simulink model "c00001M_harness"  (R2018a)
settings: Solver=ode3  StartTime=0.0  StopTime=10.0  RelTol=1e-3  EnableMultiTasking=on
undefined symbols (not defined in the file): b, DiscIntNeverNeededParam, J, K, L, R, sigbuilder_block
(part 4 of 19)

== system c00001M_harness/M084 ==
  DW1 : Inport  OutMin=0  OutMax=4  OutDataTypeStr=int8
  P1W2 : Inport  Port=2  OutMin=0  OutMax=4  OutDataTypeStr=int8
  O1 : Inport  Port=3  OutDataTypeStr=boolean
  O2 : Inport  Port=4  OutDataTypeStr=boolean
  Cyber : Subsystem
  M : Memory
  M1 : Memory
  Physical : Subsystem
  S1 : Subsystem
  S2 : Subsystem
  W1Pos : Outport
  W2Pos : Outport  Port=2
  wires:
  S2/1(SensorOut) -> M1/1
  Physical/2(W2) -> S2/1(PhyMeasure), W2Pos/1
  DW1/1 -> Cyber/3(DW1)
  M/1 -> Cyber/1(PosW1)
  M1/1 -> Cyber/2(PosW2)
  P1W2/1 -> Cyber/4(P1W2)
  Cyber/2(W2) -> Physical/2(InW2)
  Cyber/1(W1) -> Physical/1(InW1)
  O1/1 -> Cyber/5(OW1)
  O2/1 -> Cyber/6(OW2)
  Physical/1(W1) -> S1/1(PhyMeasure), W1Pos/1
  S1/1(SensorOut) -> M/1

== system c00001M_harness/M087 ==
  DW1 : Inport  OutMin=0  OutMax=4  OutDataTypeStr=int8
  P1W2 : Inport  Port=2  OutMin=0  OutMax=4  OutDataTypeStr=int8
  O1 : Inport  Port=3  OutDataTypeStr=boolean
  O2 : Inport  Port=4  OutDataTypeStr=boolean
  Cyber : Subsystem
  M : Memory
  M1 : Memory
  Physical : Subsystem
  S1 : Subsystem
  S2 : Subsystem
  W1Pos : Outport
  W2Pos : Outport  Port=2
  wires:
  S2/1(SensorOut) -> M1/1
  Physical/2(W2) -> S2/1(PhyMeasure), W2Pos/1
  DW1/1 -> Cyber/3(DW1)
  M/1 -> Cyber/1(PosW1)
  M1/1 -> Cyber/2(PosW2)
  P1W2/1 -> Cyber/4(P1W2)
  Cyber/2(W2) -> Physical/2(InW2)
  Cyber/1(W1) -> Physical/1(InW1)
  O1/1 -> Cyber/5(OW1)
  O2/1 -> Cyber/6(OW2)
  Physical/1(W1) -> S1/1(PhyMeasure), W1Pos/1
  S1/1(SensorOut) -> M/1

== system c00001M_harness/M088 ==
  DW1 : Inport  OutMin=0  OutMax=4  OutDataTypeStr=int8
  P1W2 : Inport  Port=2  OutMin=0  OutMax=4  OutDataTypeStr=int8
  O1 : Inport  Port=3  OutDataTypeStr=boolean
  O2 : Inport  Port=4  OutDataTypeStr=boolean
  Cyber : Subsystem
  M : Memory
  M1 : Memory
  Physical : Subsystem
  S1 : Subsystem
  S2 : Subsystem
  W1Pos : Outport
  W2Pos : Outport  Port=2
  wires:
  S2/1(SensorOut) -> M1/1
  Physical/2(W2) -> S2/1(PhyMeasure), W2Pos/1
  DW1/1 -> Cyber/3(DW1)
  M/1 -> Cyber/1(PosW1)
  M1/1 -> Cyber/2(PosW2)
  P1W2/1 -> Cyber/4(P1W2)
  Cyber/2(W2) -> Physical/2(InW2)
  Cyber/1(W1) -> Physical/1(InW1)
  O1/1 -> Cyber/5(OW1)
  O2/1 -> Cyber/6(OW2)
  Physical/1(W1) -> S1/1(PhyMeasure), W1Pos/1
  S1/1(SensorOut) -> M/1

== system c00001M_harness/M091 ==
  DW1 : Inport  OutMin=0  OutMax=4  OutDataTypeStr=int8
  P1W2 : Inport  Port=2  OutMin=0  OutMax=4  OutDataTypeStr=int8
  O1 : Inport  Port=3  OutDataTypeStr=boolean
  O2 : Inport  Port=4  OutDataTypeStr=boolean
  Cyber : Subsystem
  M : Memory
  M1 : Memory
  Physical : Subsystem
  S1 : Subsystem
  S2 : Subsystem
  W1Pos : Outport
  W2Pos : Outport  Port=2
  wires:
  S2/1(SensorOut) -> M1/1
  Physical/2(W2) -> S2/1(PhyMeasure), W2Pos/1
  DW1/1 -> Cyber/3(DW1)
  M/1 -> Cyber/1(PosW1)
  M1/1 -> Cyber/2(PosW2)
  P1W2/1 -> Cyber/4(P1W2)
  Cyber/2(W2) -> Physical/2(InW2)
  Cyber/1(W1) -> Physical/1(InW1)
  O1/1 -> Cyber/5(OW1)
  O2/1 -> Cyber/6(OW2)
  Physical/1(W1) -> S1/1(PhyMeasure), W1Pos/1
  S1/1(SensorOut) -> M/1

== system c00001M_harness/M092 ==
  DW1 : Inport  OutMin=0  OutMax=4  OutDataTypeStr=int8
  P1W2 : Inport  Port=2  OutMin=0  OutMax=4  OutDataTypeStr=int8
  O1 : Inport  Port=3  OutDataTypeStr=boolean
  O2 : Inport  Port=4  OutDataTypeStr=boolean
  Cyber : Subsystem
  M : Memory
  M1 : Memory
  Physical : Subsystem
  S1 : Subsystem
  S2 : Subsystem
  W1Pos : Outport
  W2Pos : Outport  Port=2
  wires:
  S2/1(SensorOut) -> M1/1
  Physical/2(W2) -> S2/1(PhyMeasure), W2Pos/1
  DW1/1 -> Cyber/3(DW1)
  M/1 -> Cyber/1(PosW1)
  M1/1 -> Cyber/2(PosW2)
  P1W2/1 -> Cyber/4(P1W2)
  Cyber/2(W2) -> Physical/2(InW2)
  Cyber/1(W1) -> Physical/1(InW1)
  O1/1 -> Cyber/5(OW1)
  O2/1 -> Cyber/6(OW2)
  Physical/1(W1) -> S1/1(PhyMeasure), W1Pos/1
  S1/1(SensorOut) -> M/1

== system c00001M_harness/M095 ==
  DW1 : Inport  OutMin=0  OutMax=4  OutDataTypeStr=int8
  P1W2 : Inport  Port=2  OutMin=0  OutMax=4  OutDataTypeStr=int8
  O1 : Inport  Port=3  OutDataTypeStr=boolean
  O2 : Inport  Port=4  OutDataTypeStr=boolean
  Cyber : Subsystem
  M : Memory
  M1 : Memory
  Physical : Subsystem
  S1 : Subsystem
  S2 : Subsystem
  W1Pos : Outport
  W2Pos : Outport  Port=2
  wires:
  S2/1(SensorOut) -> M1/1
  Physical/2(W2) -> S2/1(PhyMeasure), W2Pos/1
  DW1/1 -> Cyber/3(DW1)
  M/1 -> Cyber/1(PosW1)
  M1/1 -> Cyber/2(PosW2)
  P1W2/1 -> Cyber/4(P1W2)
  Cyber/2(W2) -> Physical/2(InW2)
  Cyber/1(W1) -> Physical/1(InW1)
  O1/1 -> Cyber/5(OW1)
  O2/1 -> Cyber/6(OW2)
  Physical/1(W1) -> S1/1(PhyMeasure), W1Pos/1
  S1/1(SensorOut) -> M/1

== system c00001M_harness/M096 ==
  DW1 : Inport  OutMin=0  OutMax=4  OutDataTypeStr=int8
  P1W2 : Inport  Port=2  OutMin=0  OutMax=4  OutDataTypeStr=int8
  O1 : Inport  Port=3  OutDataTypeStr=boolean
  O2 : Inport  Port=4  OutDataTypeStr=boolean
  Cyber : Subsystem
  M : Memory
  M1 : Memory
  Physical : Subsystem
  S1 : Subsystem
  S2 : Subsystem
  W1Pos : Outport
  W2Pos : Outport  Port=2
  wires:
  S2/1(SensorOut) -> M1/1
  Physical/2(W2) -> S2/1(PhyMeasure), W2Pos/1
  DW1/1 -> Cyber/3(DW1)
  M/1 -> Cyber/1(PosW1)
  M1/1 -> Cyber/2(PosW2)
  P1W2/1 -> Cyber/4(P1W2)
  Cyber/2(W2) -> Physical/2(InW2)
  Cyber/1(W1) -> Physical/1(InW1)
  O1/1 -> Cyber/5(OW1)
  O2/1 -> Cyber/6(OW2)
  Physical/1(W1) -> S1/1(PhyMeasure), W1Pos/1
  S1/1(SensorOut) -> M/1

== system c00001M_harness/M099 ==
  DW1 : Inport  OutMin=0  OutMax=4  OutDataTypeStr=int8
  P1W2 : Inport  Port=2  OutMin=0  OutMax=4  OutDataTypeStr=int8
  O1 : Inport  Port=3  OutDataTypeStr=boolean
  O2 : Inport  Port=4  OutDataTypeStr=boolean
  Cyber : Subsystem
  M : Memory
  M1 : Memory
  Physical : Subsystem
  S1 : Subsystem
  S2 : Subsystem
  W1Pos : Outport
  W2Pos : Outport  Port=2
  wires:
  S2/1(SensorOut) -> M1/1
  Physical/2(W2) -> S2/1(PhyMeasure), W2Pos/1
  DW1/1 -> Cyber/3(DW1)
  M/1 -> Cyber/1(PosW1)
  M1/1 -> Cyber/2(PosW2)
  P1W2/1 -> Cyber/4(P1W2)
  Cyber/2(W2) -> Physical/2(InW2)
  Cyber/1(W1) -> Physical/1(InW1)
  O1/1 -> Cyber/5(OW1)
  O2/1 -> Cyber/6(OW2)
  Physical/1(W1) -> S1/1(PhyMeasure), W1Pos/1
  S1/1(SensorOut) -> M/1

== system c00001M_harness/M100 ==
  DW1 : Inport  OutMin=0  OutMax=4  OutDataTypeStr=int8
  P1W2 : Inport  Port=2  OutMin=0  OutMax=4  OutDataTypeStr=int8
  O1 : Inport  Port=3  OutDataTypeStr=boolean
  O2 : Inport  Port=4  OutDataTypeStr=boolean
  Cyber : Subsystem
  M : Memory
  M1 : Memory
  Physical : Subsystem
  S1 : Subsystem
  S2 : Subsystem
  W1Pos : Outport
  W2Pos : Outport  Port=2
  wires:
  S2/1(SensorOut) -> M1/1
  Physical/2(W2) -> S2/1(PhyMeasure), W2Pos/1
  DW1/1 -> Cyber/3(DW1)
  M/1 -> Cyber/1(PosW1)
  M1/1 -> Cyber/2(PosW2)
  P1W2/1 -> Cyber/4(P1W2)
  Cyber/2(W2) -> Physical/2(InW2)
  Cyber/1(W1) -> Physical/1(InW1)
  O1/1 -> Cyber/5(OW1)
  O2/1 -> Cyber/6(OW2)
  Physical/1(W1) -> S1/1(PhyMeasure), W1Pos/1
  S1/1(SensorOut) -> M/1

== system c00001M_harness/M103 ==
  DW1 : Inport  OutMin=0  OutMax=4  OutDataTypeStr=int8
  P1W2 : Inport  Port=2  OutMin=0  OutMax=4  OutDataTypeStr=int8
  O1 : Inport  Port=3  OutDataTypeStr=boolean
  O2 : Inport  Port=4  OutDataTypeStr=boolean
  Cyber : Subsystem
  M : Memory
  M1 : Memory
  Physical : Subsystem
  S1 : Subsystem
  S2 : Subsystem
  W1Pos : Outport
  W2Pos : Outport  Port=2
  wires:
  S2/1(SensorOut) -> M1/1
  Physical/2(W2) -> S2/1(PhyMeasure), W2Pos/1
  DW1/1 -> Cyber/3(DW1)
  M/1 -> Cyber/1(PosW1)
  M1/1 -> Cyber/2(PosW2)
  P1W2/1 -> Cyber/4(P1W2)
  Cyber/2(W2) -> Physical/2(InW2)
  Cyber/1(W1) -> Physical/1(InW1)
  O1/1 -> Cyber/5(OW1)
  O2/1 -> Cyber/6(OW2)
  Physical/1(W1) -> S1/1(PhyMeasure), W1Pos/1
  S1/1(SensorOut) -> M/1

== system c00001M_harness/M104 ==
  DW1 : Inport  OutMin=0  OutMax=4  OutDataTypeStr=int8
  P1W2 : Inport  Port=2  OutMin=0  OutMax=4  OutDataTypeStr=int8
  O1 : Inport  Port=3  OutDataTypeStr=boolean
  O2 : Inport  Port=4  OutDataTypeStr=boolean
  Cyber : Subsystem
  M : Memory
  M1 : Memory
  Physical : Subsystem
  S1 : Subsystem
  S2 : Subsystem
  W1Pos : Outport
  W2Pos : Outport  Port=2
  wires:
  S2/1(SensorOut) -> M1/1
  Physical/2(W2) -> S2/1(PhyMeasure), W2Pos/1
  DW1/1 -> Cyber/3(DW1)
  M/1 -> Cyber/1(PosW1)
  M1/1 -> Cyber/2(PosW2)
  P1W2/1 -> Cyber/4(P1W2)
  Cyber/2(W2) -> Physical/2(InW2)
  Cyber/1(W1) -> Physical/1(InW1)
  O1/1 -> Cyber/5(OW1)
  O2/1 -> Cyber/6(OW2)
  Physical/1(W1) -> S1/1(PhyMeasure), W1Pos/1
  S1/1(SensorOut) -> M/1

== system c00001M_harness/M107 ==
  DW1 : Inport  OutMin=0  OutMax=4  OutDataTypeStr=int8
  P1W2 : Inport  Port=2  OutMin=0  OutMax=4  OutDataTypeStr=int8
  O1 : Inport  Port=3  OutDataTypeStr=boolean
  O2 : Inport  Port=4  OutDataTypeStr=boolean
  Cyber : Subsystem
  M : Memory
  M1 : Memory
  Physical : Subsystem
  S1 : Subsystem
  S2 : Subsystem
  W1Pos : Outport
  W2Pos : Outport  Port=2
  wires:
  S2/1(SensorOut) -> M1/1
  Physical/2(W2) -> S2/1(PhyMeasure), W2Pos/1
  DW1/1 -> Cyber/3(DW1)
  M/1 -> Cyber/1(PosW1)
  M1/1 -> Cyber/2(PosW2)
  P1W2/1 -> Cyber/4(P1W2)
  Cyber/2(W2) -> Physical/2(InW2)
  Cyber/1(W1) -> Physical/1(InW1)
  O1/1 -> Cyber/5(OW1)
  O2/1 -> Cyber/6(OW2)
  Physical/1(W1) -> S1/1(PhyMeasure), W1Pos/1
  S1/1(SensorOut) -> M/1

== system c00001M_harness/M108 ==
  DW1 : Inport  OutMin=0  OutMax=4  OutDataTypeStr=int8
  P1W2 : Inport  Port=2  OutMin=0  OutMax=4  OutDataTypeStr=int8
  O1 : Inport  Port=3  OutDataTypeStr=boolean
  O2 : Inport  Port=4  OutDataTypeStr=boolean
  Cyber : Subsystem
  M : Memory
  M1 : Memory
  Physical : Subsystem
  S1 : Subsystem
  S2 : Subsystem
  W1Pos : Outport
  W2Pos : Outport  Port=2
  wires:
  S2/1(SensorOut) -> M1/1
  Physical/2(W2) -> S2/1(PhyMeasure), W2Pos/1
  DW1/1 -> Cyber/3(DW1)
  M/1 -> Cyber/1(PosW1)
  M1/1 -> Cyber/2(PosW2)
  P1W2/1 -> Cyber/4(P1W2)
  Cyber/2(W2) -> Physical/2(InW2)
  Cyber/1(W1) -> Physical/1(InW1)
  O1/1 -> Cyber/5(OW1)
  O2/1 -> Cyber/6(OW2)
  Physical/1(W1) -> S1/1(PhyMeasure), W1Pos/1
  S1/1(SensorOut) -> M/1

== system c00001M_harness/M111 ==
  DW1 : Inport  OutMin=0  OutMax=4  OutDataTypeStr=int8
  P1W2 : Inport  Port=2  OutMin=0  OutMax=4  OutDataTypeStr=int8
  O1 : Inport  Port=3  OutDataTypeStr=boolean
  O2 : Inport  Port=4  OutDataTypeStr=boolean
  Cyber : Subsystem
  M : Memory
  M1 : Memory
  Physical : Subsystem
  S1 : Subsystem
  S2 : Subsystem
  W1Pos : Outport
  W2Pos : Outport  Port=2
  wires:
  S2/1(SensorOut) -> M1/1
  Physical/2(W2) -> S2/1(PhyMeasure), W2Pos/1
  DW1/1 -> Cyber/3(DW1)
  M/1 -> Cyber/1(PosW1)
  M1/1 -> Cyber/2(PosW2)
  P1W2/1 -> Cyber/4(P1W2)
  Cyber/2(W2) -> Physical/2(InW2)
  Cyber/1(W1) -> Physical/1(InW1)
  O1/1 -> Cyber/5(OW1)
  O2/1 -> Cyber/6(OW2)
  Physical/1(W1) -> S1/1(PhyMeasure), W1Pos/1
  S1/1(SensorOut) -> M/1

== system c00001M_harness/M112 ==
  DW1 : Inport  OutMin=0  OutMax=4  OutDataTypeStr=int8
  P1W2 : Inport  Port=2  OutMin=0  OutMax=4  OutDataTypeStr=int8
  O1 : Inport  Port=3  OutDataTypeStr=boolean
  O2 : Inport  Port=4  OutDataTypeStr=boolean
  Cyber : Subsystem
  M : Memory
  M1 : Memory
  Physical : Subsystem
  S1 : Subsystem
  S2 : Subsystem
  W1Pos : Outport
  W2Pos : Outport  Port=2
  wires:
  S2/1(SensorOut) -> M1/1
  Physical/2(W2) -> S2/1(PhyMeasure), W2Pos/1
  DW1/1 -> Cyber/3(DW1)
  M/1 -> Cyber/1(PosW1)
  M1/1 -> Cyber/2(PosW2)
  P1W2/1 -> Cyber/4(P1W2)
  Cyber/2(W2) -> Physical/2(InW2)
  Cyber/1(W1) -> Physical/1(InW1)
  O1/1 -> Cyber/5(OW1)
  O2/1 -> Cyber/6(OW2)
  Physical/1(W1) -> S1/1(PhyMeasure), W1Pos/1
  S1/1(SensorOut) -> M/1

== system c00001M_harness/M115 ==
  DW1 : Inport  OutMin=0  OutMax=4  OutDataTypeStr=int8
  P1W2 : Inport  Port=2  OutMin=0  OutMax=4  OutDataTypeStr=int8
  O1 : Inport  Port=3  OutDataTypeStr=boolean
  O2 : Inport  Port=4  OutDataTypeStr=boolean
  Cyber : Subsystem
  M : Memory
  M1 : Memory
  Physical : Subsystem
  S1 : Subsystem
  S2 : Subsystem
  W1Pos : Outport
  W2Pos : Outport  Port=2
  wires:
  S2/1(SensorOut) -> M1/1
  Physical/2(W2) -> S2/1(PhyMeasure), W2Pos/1
  DW1/1 -> Cyber/3(DW1)
  M/1 -> Cyber/1(PosW1)
  M1/1 -> Cyber/2(PosW2)
  P1W2/1 -> Cyber/4(P1W2)
  Cyber/2(W2) -> Physical/2(InW2)
  Cyber/1(W1) -> Physical/1(InW1)
  O1/1 -> Cyber/5(OW1)
  O2/1 -> Cyber/6(OW2)
  Physical/1(W1) -> S1/1(PhyMeasure), W1Pos/1
  S1/1(SensorOut) -> M/1

== system c00001M_harness/M116 ==
  DW1 : Inport  OutMin=0  OutMax=4  OutDataTypeStr=int8
  P1W2 : Inport  Port=2  OutMin=0  OutMax=4  OutDataTypeStr=int8
  O1 : Inport  Port=3  OutDataTypeStr=boolean
  O2 : Inport  Port=4  OutDataTypeStr=boolean
  Cyber : Subsystem
  M : Memory
  M1 : Memory
  Physical : Subsystem
  S1 : Subsystem
  S2 : Subsystem
  W1Pos : Outport
  W2Pos : Outport  Port=2
  wires:
  S2/1(SensorOut) -> M1/1
  Physical/2(W2) -> S2/1(PhyMeasure), W2Pos/1
  DW1/1 -> Cyber/3(DW1)
  M/1 -> Cyber/1(PosW1)
  M1/1 -> Cyber/2(PosW2)
  P1W2/1 -> Cyber/4(P1W2)
  Cyber/2(W2) -> Physical/2(InW2)
  Cyber/1(W1) -> Physical/1(InW1)
  O1/1 -> Cyber/5(OW1)
  O2/1 -> Cyber/6(OW2)
  Physical/1(W1) -> S1/1(PhyMeasure), W1Pos/1
  S1/1(SensorOut) -> M/1

== system c00001M_harness/M119 ==
  DW1 : Inport  OutMin=0  OutMax=4  OutDataTypeStr=int8
  P1W2 : Inport  Port=2  OutMin=0  OutMax=4  OutDataTypeStr=int8
  O1 : Inport  Port=3  OutDataTypeStr=boolean
  O2 : Inport  Port=4  OutDataTypeStr=boolean
  Cyber : Subsystem
  M : Memory
  M1 : Memory
  Physical : Subsystem
  S1 : Subsystem
  S2 : Subsystem
  W1Pos : Outport
  W2Pos : Outport  Port=2
  wires:
  S2/1(SensorOut) -> M1/1
  Physical/2(W2) -> S2/1(PhyMeasure), W2Pos/1
  DW1/1 -> Cyber/3(DW1)
  M/1 -> Cyber/1(PosW1)
  M1/1 -> Cyber/2(PosW2)
  P1W2/1 -> Cyber/4(P1W2)
  Cyber/2(W2) -> Physical/2(InW2)
  Cyber/1(W1) -> Physical/1(InW1)
  O1/1 -> Cyber/5(OW1)
  O2/1 -> Cyber/6(OW2)
  Physical/1(W1) -> S1/1(PhyMeasure), W1Pos/1
  S1/1(SensorOut) -> M/1

== system c00001M_harness/M120 ==
  DW1 : Inport  OutMin=0  OutMax=4  OutDataTypeStr=int8
  P1W2 : Inport  Port=2  OutMin=0  OutMax=4  OutDataTypeStr=int8
  O1 : Inport  Port=3  OutDataTypeStr=boolean
  O2 : Inport  Port=4  OutDataTypeStr=boolean
  Cyber : Subsystem
  M : Memory
  M1 : Memory
  Physical : Subsystem
  S1 : Subsystem
  S2 : Subsystem
  W1Pos : Outport
  W2Pos : Outport  Port=2
  wires:
  S2/1(SensorOut) -> M1/1
  Physical/2(W2) -> S2/1(PhyMeasure), W2Pos/1
  DW1/1 -> Cyber/3(DW1)
  M/1 -> Cyber/1(PosW1)
  M1/1 -> Cyber/2(PosW2)
  P1W2/1 -> Cyber/4(P1W2)
  Cyber/2(W2) -> Physical/2(InW2)
  Cyber/1(W1) -> Physical/1(InW1)
  O1/1 -> Cyber/5(OW1)
  O2/1 -> Cyber/6(OW2)
  Physical/1(W1) -> S1/1(PhyMeasure), W1Pos/1
  S1/1(SensorOut) -> M/1

== system c00001M_harness/M123 ==
  DW1 : Inport  OutMin=0  OutMax=4  OutDataTypeStr=int8
  P1W2 : Inport  Port=2  OutMin=0  OutMax=4  OutDataTypeStr=int8
  O1 : Inport  Port=3  OutDataTypeStr=boolean
  O2 : Inport  Port=4  OutDataTypeStr=boolean
  Cyber : Subsystem
  M : Memory
  M1 : Memory
  Physical : Subsystem
  S1 : Subsystem
  S2 : Subsystem
  W1Pos : Outport
  W2Pos : Outport  Port=2
  wires:
  S2/1(SensorOut) -> M1/1
  Physical/2(W2) -> S2/1(PhyMeasure), W2Pos/1
  DW1/1 -> Cyber/3(DW1)
  M/1 -> Cyber/1(PosW1)
  M1/1 -> Cyber/2(PosW2)
  P1W2/1 -> Cyber/4(P1W2)
  Cyber/2(W2) -> Physical/2(InW2)
  Cyber/1(W1) -> Physical/1(InW1)
  O1/1 -> Cyber/5(OW1)
  O2/1 -> Cyber/6(OW2)
  Physical/1(W1) -> S1/1(PhyMeasure), W1Pos/1
  S1/1(SensorOut) -> M/1

== system c00001M_harness/M124 ==
  DW1 : Inport  OutMin=0  OutMax=4  OutDataTypeStr=int8
  P1W2 : Inport  Port=2  OutMin=0  OutMax=4  OutDataTypeStr=int8
  O1 : Inport  Port=3  OutDataTypeStr=boolean
  O2 : Inport  Port=4  OutDataTypeStr=boolean
  Cyber : Subsystem
  M : Memory
  M1 : Memory
  Physical : Subsystem
  S1 : Subsystem
  S2 : Subsystem
  W1Pos : Outport
  W2Pos : Outport  Port=2
  wires:
  S2/1(SensorOut) -> M1/1
  Physical/2(W2) -> S2/1(PhyMeasure), W2Pos/1
  DW1/1 -> Cyber/3(DW1)
  M/1 -> Cyber/1(PosW1)
  M1/1 -> Cyber/2(PosW2)
  P1W2/1 -> Cyber/4(P1W2)
  Cyber/2(W2) -> Physical/2(InW2)
  Cyber/1(W1) -> Physical/1(InW1)
  O1/1 -> Cyber/5(OW1)
  O2/1 -> Cyber/6(OW2)
  Physical/1(W1) -> S1/1(PhyMeasure), W1Pos/1
  S1/1(SensorOut) -> M/1

== system c00001M_harness/M127 ==
  DW1 : Inport  OutMin=0  OutMax=4  OutDataTypeStr=int8
  P1W2 : Inport  Port=2  OutMin=0  OutMax=4  OutDataTypeStr=int8
  O1 : Inport  Port=3  OutDataTypeStr=boolean
  O2 : Inport  Port=4  OutDataTypeStr=boolean
  Cyber : Subsystem
  M : Memory
  M1 : Memory
  Physical : Subsystem
  S1 : Subsystem
  S2 : Subsystem
  W1Pos : Outport
  W2Pos : Outport  Port=2
  wires:
  S2/1(SensorOut) -> M1/1
  Physical/2(W2) -> S2/1(PhyMeasure), W2Pos/1
  DW1/1 -> Cyber/3(DW1)
  M/1 -> Cyber/1(PosW1)
  M1/1 -> Cyber/2(PosW2)
  P1W2/1 -> Cyber/4(P1W2)
  Cyber/2(W2) -> Physical/2(InW2)
  Cyber/1(W1) -> Physical/1(InW1)
  O1/1 -> Cyber/5(OW1)
  O2/1 -> Cyber/6(OW2)
  Physical/1(W1) -> S1/1(PhyMeasure), W1Pos/1
  S1/1(SensorOut) -> M/1

== system c00001M_harness/M128 ==
  DW1 : Inport  OutMin=0  OutMax=4  OutDataTypeStr=int8
  P1W2 : Inport  Port=2  OutMin=0  OutMax=4  OutDataTypeStr=int8
  O1 : Inport  Port=3  OutDataTypeStr=boolean
  O2 : Inport  Port=4  OutDataTypeStr=boolean
  Cyber : Subsystem
  M : Memory
  M1 : Memory
  Physical : Subsystem
  S1 : Subsystem
  S2 : Subsystem
  W1Pos : Outport
  W2Pos : Outport  Port=2
  wires:
  S2/1(SensorOut) -> M1/1
  Physical/2(W2) -> S2/1(PhyMeasure), W2Pos/1
  DW1/1 -> Cyber/3(DW1)
  M/1 -> Cyber/1(PosW1)
  M1/1 -> Cyber/2(PosW2)
  P1W2/1 -> Cyber/4(P1W2)
  Cyber/2(W2) -> Physical/2(InW2)
  Cyber/1(W1) -> Physical/1(InW1)
  O1/1 -> Cyber/5(OW1)
  O2/1 -> Cyber/6(OW2)
  Physical/1(W1) -> S1/1(PhyMeasure), W1Pos/1
  S1/1(SensorOut) -> M/1

== system c00001M_harness/M131 ==
  DW1 : Inport  OutMin=0  OutMax=4  OutDataTypeStr=int8
  P1W2 : Inport  Port=2  OutMin=0  OutMax=4  OutDataTypeStr=int8
  O1 : Inport  Port=3  OutDataTypeStr=boolean
  O2 : Inport  Port=4  OutDataTypeStr=boolean
  Cyber : Subsystem
  M : Memory
  M1 : Memory
  Physical : Subsystem
  S1 : Subsystem
  S2 : Subsystem
  W1Pos : Outport
  W2Pos : Outport  Port=2
  wires:
  S2/1(SensorOut) -> M1/1
  Physical/2(W2) -> S2/1(PhyMeasure), W2Pos/1
  DW1/1 -> Cyber/3(DW1)
  M/1 -> Cyber/1(PosW1)
  M1/1 -> Cyber/2(PosW2)
  P1W2/1 -> Cyber/4(P1W2)
  Cyber/2(W2) -> Physical/2(InW2)
  Cyber/1(W1) -> Physical/1(InW1)
  O1/1 -> Cyber/5(OW1)
  O2/1 -> Cyber/6(OW2)
  Physical/1(W1) -> S1/1(PhyMeasure), W1Pos/1
  S1/1(SensorOut) -> M/1

== system c00001M_harness/M132 ==
  DW1 : Inport  OutMin=0  OutMax=4  OutDataTypeStr=int8
  P1W2 : Inport  Port=2  OutMin=0  OutMax=4  OutDataTypeStr=int8
  O1 : Inport  Port=3  OutDataTypeStr=boolean
  O2 : Inport  Port=4  OutDataTypeStr=boolean
  Cyber : Subsystem
  M : Memory
  M1 : Memory
  Physical : Subsystem
  S1 : Subsystem
  S2 : Subsystem
  W1Pos : Outport
  W2Pos : Outport  Port=2
  wires:
  S2/1(SensorOut) -> M1/1
  Physical/2(W2) -> S2/1(PhyMeasure), W2Pos/1
  DW1/1 -> Cyber/3(DW1)
  M/1 -> Cyber/1(PosW1)
  M1/1 -> Cyber/2(PosW2)
  P1W2/1 -> Cyber/4(P1W2)
  Cyber/2(W2) -> Physical/2(InW2)
  Cyber/1(W1) -> Physical/1(InW1)
  O1/1 -> Cyber/5(OW1)
  O2/1 -> Cyber/6(OW2)
  Physical/1(W1) -> S1/1(PhyMeasure), W1Pos/1
  S1/1(SensorOut) -> M/1

== system c00001M_harness/M135 ==
  DW1 : Inport  OutMin=0  OutMax=4  OutDataTypeStr=int8
  P1W2 : Inport  Port=2  OutMin=0  OutMax=4  OutDataTypeStr=int8
  O1 : Inport  Port=3  OutDataTypeStr=boolean
  O2 : Inport  Port=4  OutDataTypeStr=boolean
  Cyber : Subsystem
  M : Memory
  M1 : Memory
  Physical : Subsystem
  S1 : Subsystem
  S2 : Subsystem
  W1Pos : Outport
  W2Pos : Outport  Port=2
  wires:
  S2/1(SensorOut) -> M1/1
  Physical/2(W2) -> S2/1(PhyMeasure), W2Pos/1
  DW1/1 -> Cyber/3(DW1)
  M/1 -> Cyber/1(PosW1)
  M1/1 -> Cyber/2(PosW2)
  P1W2/1 -> Cyber/4(P1W2)
  Cyber/2(W2) -> Physical/2(InW2)
  Cyber/1(W1) -> Physical/1(InW1)
  O1/1 -> Cyber/5(OW1)
  O2/1 -> Cyber/6(OW2)
  Physical/1(W1) -> S1/1(PhyMeasure), W1Pos/1
  S1/1(SensorOut) -> M/1

== system c00001M_harness/M136 ==
  DW1 : Inport  OutMin=0  OutMax=4  OutDataTypeStr=int8
  P1W2 : Inport  Port=2  OutMin=0  OutMax=4  OutDataTypeStr=int8
  O1 : Inport  Port=3  OutDataTypeStr=boolean
  O2 : Inport  Port=4  OutDataTypeStr=boolean
  Cyber : Subsystem
  M : Memory
  M1 : Memory
  Physical : Subsystem
  S1 : Subsystem
  S2 : Subsystem
  W1Pos : Outport
  W2Pos : Outport  Port=2
  wires:
  S2/1(SensorOut) -> M1/1
  Physical/2(W2) -> S2/1(PhyMeasure), W2Pos/1
  DW1/1 -> Cyber/3(DW1)
  M/1 -> Cyber/1(PosW1)
  M1/1 -> Cyber/2(PosW2)
  P1W2/1 -> Cyber/4(P1W2)
  Cyber/2(W2) -> Physical/2(InW2)
  Cyber/1(W1) -> Physical/1(InW1)
  O1/1 -> Cyber/5(OW1)
  O2/1 -> Cyber/6(OW2)
  Physical/1(W1) -> S1/1(PhyMeasure), W1Pos/1
  S1/1(SensorOut) -> M/1

== system c00001M_harness/M139 ==
  DW1 : Inport  OutMin=0  OutMax=4  OutDataTypeStr=int8
  P1W2 : Inport  Port=2  OutMin=0  OutMax=4  OutDataTypeStr=int8
  O1 : Inport  Port=3  OutDataTypeStr=boolean
  O2 : Inport  Port=4  OutDataTypeStr=boolean
  Cyber : Subsystem
  M : Memory
  M1 : Memory
  Physical : Subsystem
  S1 : Subsystem
  S2 : Subsystem
  W1Pos : Outport
  W2Pos : Outport  Port=2
  wires:
  S2/1(SensorOut) -> M1/1
  Physical/2(W2) -> S2/1(PhyMeasure), W2Pos/1
  DW1/1 -> Cyber/3(DW1)
  M/1 -> Cyber/1(PosW1)
  M1/1 -> Cyber/2(PosW2)
  P1W2/1 -> Cyber/4(P1W2)
  Cyber/2(W2) -> Physical/2(InW2)
  Cyber/1(W1) -> Physical/1(InW1)
  O1/1 -> Cyber/5(OW1)
  O2/1 -> Cyber/6(OW2)
  Physical/1(W1) -> S1/1(PhyMeasure), W1Pos/1
  S1/1(SensorOut) -> M/1

== system c00001M_harness/M140 ==
  DW1 : Inport  OutMin=0  OutMax=4  OutDataTypeStr=int8
  P1W2 : Inport  Port=2  OutMin=0  OutMax=4  OutDataTypeStr=int8
  O1 : Inport  Port=3  OutDataTypeStr=boolean
  O2 : Inport  Port=4  OutDataTypeStr=boolean
  Cyber : Subsystem
  M : Memory
  M1 : Memory
  Physical : Subsystem
  S1 : Subsystem
  S2 : Subsystem
  W1Pos : Outport
  W2Pos : Outport  Port=2
  wires:
  S2/1(SensorOut) -> M1/1
  Physical/2(W2) -> S2/1(PhyMeasure), W2Pos/1
  DW1/1 -> Cyber/3(DW1)
  M/1 -> Cyber/1(PosW1)
  M1/1 -> Cyber/2(PosW2)
  P1W2/1 -> Cyber/4(P1W2)
  Cyber/2(W2) -> Physical/2(InW2)
  Cyber/1(W1) -> Physical/1(InW1)
  O1/1 -> Cyber/5(OW1)
  O2/1 -> Cyber/6(OW2)
  Physical/1(W1) -> S1/1(PhyMeasure), W1Pos/1
  S1/1(SensorOut) -> M/1

== system c00001M_harness/M143 ==
  DW1 : Inport  OutMin=0  OutMax=4  OutDataTypeStr=int8
  P1W2 : Inport  Port=2  OutMin=0  OutMax=4  OutDataTypeStr=int8
  O1 : Inport  Port=3  OutDataTypeStr=boolean
  O2 : Inport  Port=4  OutDataTypeStr=boolean
  Cyber : Subsystem
  M : Memory
  M1 : Memory
  Physical : Subsystem
  S1 : Subsystem
  S2 : Subsystem
  W1Pos : Outport
  W2Pos : Outport  Port=2
  wires:
  S2/1(SensorOut) -> M1/1
  Physical/2(W2) -> S2/1(PhyMeasure), W2Pos/1
  DW1/1 -> Cyber/3(DW1)
  M/1 -> Cyber/1(PosW1)
  M1/1 -> Cyber/2(PosW2)
  P1W2/1 -> Cyber/4(P1W2)
  Cyber/2(W2) -> Physical/2(InW2)
  Cyber/1(W1) -> Physical/1(InW1)
  O1/1 -> Cyber/5(OW1)
  O2/1 -> Cyber/6(OW2)
  Physical/1(W1) -> S1/1(PhyMeasure), W1Pos/1
  S1/1(SensorOut) -> M/1

== system c00001M_harness/M144 ==
  DW1 : Inport  OutMin=0  OutMax=4  OutDataTypeStr=int8
  P1W2 : Inport  Port=2  OutMin=0  OutMax=4  OutDataTypeStr=int8
  O1 : Inport  Port=3  OutDataTypeStr=boolean
  O2 : Inport  Port=4  OutDataTypeStr=boolean
  Cyber : Subsystem
  M : Memory
  M1 : Memory
  Physical : Subsystem
  S1 : Subsystem
  S2 : Subsystem
  W1Pos : Outport
  W2Pos : Outport  Port=2
  wires:
  S2/1(SensorOut) -> M1/1
  Physical/2(W2) -> S2/1(PhyMeasure), W2Pos/1
  DW1/1 -> Cyber/3(DW1)
  M/1 -> Cyber/1(PosW1)
  M1/1 -> Cyber/2(PosW2)
  P1W2/1 -> Cyber/4(P1W2)
  Cyber/2(W2) -> Physical/2(InW2)
  Cyber/1(W1) -> Physical/1(InW1)
  O1/1 -> Cyber/5(OW1)
  O2/1 -> Cyber/6(OW2)
  Physical/1(W1) -> S1/1(PhyMeasure), W1Pos/1
  S1/1(SensorOut) -> M/1

== system c00001M_harness/M147 ==
  DW1 : Inport  OutMin=0  OutMax=4  OutDataTypeStr=int8
  P1W2 : Inport  Port=2  OutMin=0  OutMax=4  OutDataTypeStr=int8
  O1 : Inport  Port=3  OutDataTypeStr=boolean
  O2 : Inport  Port=4  OutDataTypeStr=boolean
  Cyber : Subsystem
  M : Memory
  M1 : Memory
  Physical : Subsystem
  S1 : Subsystem
  S2 : Subsystem
  W1Pos : Outport
  W2Pos : Outport  Port=2
  wires:
  S2/1(SensorOut) -> M1/1
  Physical/2(W2) -> S2/1(PhyMeasure), W2Pos/1
  DW1/1 -> Cyber/3(DW1)
  M/1 -> Cyber/1(PosW1)
  M1/1 -> Cyber/2(PosW2)
  P1W2/1 -> Cyber/4(P1W2)
  Cyber/2(W2) -> Physical/2(InW2)
  Cyber/1(W1) -> Physical/1(InW1)
  O1/1 -> Cyber/5(OW1)
  O2/1 -> Cyber/6(OW2)
  Physical/1(W1) -> S1/1(PhyMeasure), W1Pos/1
  S1/1(SensorOut) -> M/1

== system c00001M_harness/M148 ==
  DW1 : Inport  OutMin=0  OutMax=4  OutDataTypeStr=int8
  P1W2 : Inport  Port=2  OutMin=0  OutMax=4  OutDataTypeStr=int8
  O1 : Inport  Port=3  OutDataTypeStr=boolean
  O2 : Inport  Port=4  OutDataTypeStr=boolean
  Cyber : Subsystem
  M : Memory
  M1 : Memory
  Physical : Subsystem
  S1 : Subsystem
  S2 : Subsystem
  W1Pos : Outport
  W2Pos : Outport  Port=2
  wires:
  S2/1(SensorOut) -> M1/1
  Physical/2(W2) -> S2/1(PhyMeasure), W2Pos/1
  DW1/1 -> Cyber/3(DW1)
  M/1 -> Cyber/1(PosW1)
  M1/1 -> Cyber/2(PosW2)
  P1W2/1 -> Cyber/4(P1W2)
  Cyber/2(W2) -> Physical/2(InW2)
  Cyber/1(W1) -> Physical/1(InW1)
  O1/1 -> Cyber/5(OW1)
  O2/1 -> Cyber/6(OW2)
  Physical/1(W1) -> S1/1(PhyMeasure), W1Pos/1
  S1/1(SensorOut) -> M/1

== system c00001M_harness/M151 ==
  DW1 : Inport  OutMin=0  OutMax=4  OutDataTypeStr=int8
  P1W2 : Inport  Port=2  OutMin=0  OutMax=4  OutDataTypeStr=int8
  O1 : Inport  Port=3  OutDataTypeStr=boolean
  O2 : Inport  Port=4  OutDataTypeStr=boolean
  Cyber : Subsystem
  M : Memory
  M1 : Memory
  Physical : Subsystem
  S1 : Subsystem
  S2 : Subsystem
  W1Pos : Outport
  W2Pos : Outport  Port=2
  wires:
  S2/1(SensorOut) -> M1/1
  Physical/2(W2) -> S2/1(PhyMeasure), W2Pos/1
  DW1/1 -> Cyber/3(DW1)
  M/1 -> Cyber/1(PosW1)
  M1/1 -> Cyber/2(PosW2)
  P1W2/1 -> Cyber/4(P1W2)
  Cyber/2(W2) -> Physical/2(InW2)
  Cyber/1(W1) -> Physical/1(InW1)
  O1/1 -> Cyber/5(OW1)
  O2/1 -> Cyber/6(OW2)
  Physical/1(W1) -> S1/1(PhyMeasure), W1Pos/1
  S1/1(SensorOut) -> M/1

== system c00001M_harness/M152 ==
  DW1 : Inport  OutMin=0  OutMax=4  OutDataTypeStr=int8
  P1W2 : Inport  Port=2  OutMin=0  OutMax=4  OutDataTypeStr=int8
  O1 : Inport  Port=3  OutDataTypeStr=boolean
  O2 : Inport  Port=4  OutDataTypeStr=boolean
  Cyber : Subsystem
  M : Memory
  M1 : Memory
  Physical : Subsystem
  S1 : Subsystem
  S2 : Subsystem
  W1Pos : Outport
  W2Pos : Outport  Port=2
  wires:
  S2/1(SensorOut) -> M1/1
  Physical/2(W2) -> S2/1(PhyMeasure), W2Pos/1
  DW1/1 -> Cyber/3(DW1)
  M/1 -> Cyber/1(PosW1)
  M1/1 -> Cyber/2(PosW2)
  P1W2/1 -> Cyber/4(P1W2)
  Cyber/2(W2) -> Physical/2(InW2)
  Cyber/1(W1) -> Physical/1(InW1)
  O1/1 -> Cyber/5(OW1)
  O2/1 -> Cyber/6(OW2)
  Physical/1(W1) -> S1/1(PhyMeasure), W1Pos/1
  S1/1(SensorOut) -> M/1

== system c00001M_harness/M155 ==
  DW1 : Inport  OutMin=0  OutMax=4  OutDataTypeStr=int8
  P1W2 : Inport  Port=2  OutMin=0  OutMax=4  OutDataTypeStr=int8
  O1 : Inport  Port=3  OutDataTypeStr=boolean
  O2 : Inport  Port=4  OutDataTypeStr=boolean
  Cyber : Subsystem
  M : Memory
  M1 : Memory
  Physical : Subsystem
  S1 : Subsystem
  S2 : Subsystem
  W1Pos : Outport
  W2Pos : Outport  Port=2
  wires:
  S2/1(SensorOut) -> M1/1
  Physical/2(W2) -> S2/1(PhyMeasure), W2Pos/1
  DW1/1 -> Cyber/3(DW1)
  M/1 -> Cyber/1(PosW1)
  M1/1 -> Cyber/2(PosW2)
  P1W2/1 -> Cyber/4(P1W2)
  Cyber/2(W2) -> Physical/2(InW2)
  Cyber/1(W1) -> Physical/1(InW1)
  O1/1 -> Cyber/5(OW1)
  O2/1 -> Cyber/6(OW2)
  Physical/1(W1) -> S1/1(PhyMeasure), W1Pos/1
  S1/1(SensorOut) -> M/1

== system c00001M_harness/M156 ==
  DW1 : Inport  OutMin=0  OutMax=4  OutDataTypeStr=int8
  P1W2 : Inport  Port=2  OutMin=0  OutMax=4  OutDataTypeStr=int8
  O1 : Inport  Port=3  OutDataTypeStr=boolean
  O2 : Inport  Port=4  OutDataTypeStr=boolean
  Cyber : Subsystem
  M : Memory
  M1 : Memory
  Physical : Subsystem
  S1 : Subsystem
  S2 : Subsystem
  W1Pos : Outport
  W2Pos : Outport  Port=2
  wires:
  S2/1(SensorOut) -> M1/1
  Physical/2(W2) -> S2/1(PhyMeasure), W2Pos/1
  DW1/1 -> Cyber/3(DW1)
  M/1 -> Cyber/1(PosW1)
  M1/1 -> Cyber/2(PosW2)
  P1W2/1 -> Cyber/4(P1W2)
  Cyber/2(W2) -> Physical/2(InW2)
  Cyber/1(W1) -> Physical/1(InW1)
  O1/1 -> Cyber/5(OW1)
  O2/1 -> Cyber/6(OW2)
  Physical/1(W1) -> S1/1(PhyMeasure), W1Pos/1
  S1/1(SensorOut) -> M/1

== system c00001M_harness/M159 ==
  DW1 : Inport  OutMin=0  OutMax=4  OutDataTypeStr=int8
  P1W2 : Inport  Port=2  OutMin=0  OutMax=4  OutDataTypeStr=int8
  O1 : Inport  Port=3  OutDataTypeStr=boolean
  O2 : Inport  Port=4  OutDataTypeStr=boolean
  Cyber : Subsystem
  M : Memory
  M1 : Memory
  Physical : Subsystem
  S1 : Subsystem
  S2 : Subsystem
  W1Pos : Outport
  W2Pos : Outport  Port=2
  wires:
  S2/1(SensorOut) -> M1/1
  Physical/2(W2) -> S2/1(PhyMeasure), W2Pos/1
  DW1/1 -> Cyber/3(DW1)
  M/1 -> Cyber/1(PosW1)
  M1/1 -> Cyber/2(PosW2)
  P1W2/1 -> Cyber/4(P1W2)
  Cyber/2(W2) -> Physical/2(InW2)
  Cyber/1(W1) -> Physical/1(InW1)
  O1/1 -> Cyber/5(OW1)
  O2/1 -> Cyber/6(OW2)
  Physical/1(W1) -> S1/1(PhyMeasure), W1Pos/1
  S1/1(SensorOut) -> M/1

== system c00001M_harness/M160 ==
  DW1 : Inport  OutMin=0  OutMax=4  OutDataTypeStr=int8
  P1W2 : Inport  Port=2  OutMin=0  OutMax=4  OutDataTypeStr=int8
  O1 : Inport  Port=3  OutDataTypeStr=boolean
  O2 : Inport  Port=4  OutDataTypeStr=boolean
  Cyber : Subsystem
  M : Memory
  M1 : Memory
  Physical : Subsystem
  S1 : Subsystem
  S2 : Subsystem
  W1Pos : Outport
  W2Pos : Outport  Port=2
  wires:
  S2/1(SensorOut) -> M1/1
  Physical/2(W2) -> S2/1(PhyMeasure), W2Pos/1
  DW1/1 -> Cyber/3(DW1)
  M/1 -> Cyber/1(PosW1)
  M1/1 -> Cyber/2(PosW2)
  P1W2/1 -> Cyber/4(P1W2)
  Cyber/2(W2) -> Physical/2(InW2)
  Cyber/1(W1) -> Physical/1(InW1)
  O1/1 -> Cyber/5(OW1)
  O2/1 -> Cyber/6(OW2)
  Physical/1(W1) -> S1/1(PhyMeasure), W1Pos/1
  S1/1(SensorOut) -> M/1

== system c00001M_harness/M163 ==
  DW1 : Inport  OutMin=0  OutMax=4  OutDataTypeStr=int8
  P1W2 : Inport  Port=2  OutMin=0  OutMax=4  OutDataTypeStr=int8
  O1 : Inport  Port=3  OutDataTypeStr=boolean
  O2 : Inport  Port=4  OutDataTypeStr=boolean
  Cyber : Subsystem
  M : Memory
  M1 : Memory
  Physical : Subsystem
  S1 : Subsystem
  S2 : Subsystem
  W1Pos : Outport
  W2Pos : Outport  Port=2
  wires:
  S2/1(SensorOut) -> M1/1
  Physical/2(W2) -> S2/1(PhyMeasure), W2Pos/1
  DW1/1 -> Cyber/3(DW1)
  M/1 -> Cyber/1(PosW1)
  M1/1 -> Cyber/2(PosW2)
  P1W2/1 -> Cyber/4(P1W2)
  Cyber/2(W2) -> Physical/2(InW2)
  Cyber/1(W1) -> Physical/1(InW1)
  O1/1 -> Cyber/5(OW1)
  O2/1 -> Cyber/6(OW2)
  Physical/1(W1) -> S1/1(PhyMeasure), W1Pos/1
  S1/1(SensorOut) -> M/1

== system c00001M_harness/M164 ==
  DW1 : Inport  OutMin=0  OutMax=4  OutDataTypeStr=int8
  P1W2 : Inport  Port=2  OutMin=0  OutMax=4  OutDataTypeStr=int8
  O1 : Inport  Port=3  OutDataTypeStr=boolean
  O2 : Inport  Port=4  OutDataTypeStr=boolean
  Cyber : Subsystem
  M : Memory
  M1 : Memory
  Physical : Subsystem
  S1 : Subsystem
  S2 : Subsystem
  W1Pos : Outport
  W2Pos : Outport  Port=2
  wires:
  S2/1(SensorOut) -> M1/1
  Physical/2(W2) -> S2/1(PhyMeasure), W2Pos/1
  DW1/1 -> Cyber/3(DW1)
  M/1 -> Cyber/1(PosW1)
  M1/1 -> Cyber/2(PosW2)
  P1W2/1 -> Cyber/4(P1W2)
  Cyber/2(W2) -> Physical/2(InW2)
  Cyber/1(W1) -> Physical/1(InW1)
  O1/1 -> Cyber/5(OW1)
  O2/1 -> Cyber/6(OW2)
  Physical/1(W1) -> S1/1(PhyMeasure), W1Pos/1
  S1/1(SensorOut) -> M/1

== system c00001M_harness/M167 ==
  DW1 : Inport  OutMin=0  OutMax=4  OutDataTypeStr=int8
  P1W2 : Inport  Port=2  OutMin=0  OutMax=4  OutDataTypeStr=int8
  O1 : Inport  Port=3  OutDataTypeStr=boolean
  O2 : Inport  Port=4  OutDataTypeStr=boolean
  Cyber : Subsystem
  M : Memory
  M1 : Memory
  Physical : Subsystem
  S1 : Subsystem
  S2 : Subsystem
  W1Pos : Outport
  W2Pos : Outport  Port=2
  wires:
  S2/1(SensorOut) -> M1/1
  Physical/2(W2) -> S2/1(PhyMeasure), W2Pos/1
  DW1/1 -> Cyber/3(DW1)
  M/1 -> Cyber/1(PosW1)
  M1/1 -> Cyber/2(PosW2)
  P1W2/1 -> Cyber/4(P1W2)
  Cyber/2(W2) -> Physical/2(InW2)
  Cyber/1(W1) -> Physical/1(InW1)
  O1/1 -> Cyber/5(OW1)
  O2/1 -> Cyber/6(OW2)
  Physical/1(W1) -> S1/1(PhyMeasure), W1Pos/1
  S1/1(SensorOut) -> M/1

== system c00001M_harness/M168 ==
  DW1 : Inport  OutMin=0  OutMax=4  OutDataTypeStr=int8
  P1W2 : Inport  Port=2  OutMin=0  OutMax=4  OutDataTypeStr=int8
  O1 : Inport  Port=3  OutDataTypeStr=boolean
  O2 : Inport  Port=4  OutDataTypeStr=boolean
  Cyber : Subsystem
  M : Memory
  M1 : Memory
  Physical : Subsystem
  S1 : Subsystem
  S2 : Subsystem
  W1Pos : Outport
  W2Pos : Outport  Port=2
  wires:
  S2/1(SensorOut) -> M1/1
  Physical/2(W2) -> S2/1(PhyMeasure), W2Pos/1
  DW1/1 -> Cyber/3(DW1)
  M/1 -> Cyber/1(PosW1)
  M1/1 -> Cyber/2(PosW2)
  P1W2/1 -> Cyber/4(P1W2)
  Cyber/2(W2) -> Physical/2(InW2)
  Cyber/1(W1) -> Physical/1(InW1)
  O1/1 -> Cyber/5(OW1)
  O2/1 -> Cyber/6(OW2)
  Physical/1(W1) -> S1/1(PhyMeasure), W1Pos/1
  S1/1(SensorOut) -> M/1

== system c00001M_harness/M171 ==
  DW1 : Inport  OutMin=0  OutMax=4  OutDataTypeStr=int8
  P1W2 : Inport  Port=2  OutMin=0  OutMax=4  OutDataTypeStr=int8
  O1 : Inport  Port=3  OutDataTypeStr=boolean
  O2 : Inport  Port=4  OutDataTypeStr=boolean
  Cyber : Subsystem
  M : Memory
  M1 : Memory
  Physical : Subsystem
  S1 : Subsystem
  S2 : Subsystem
  W1Pos : Outport
  W2Pos : Outport  Port=2
  wires:
  S2/1(SensorOut) -> M1/1
  Physical/2(W2) -> S2/1(PhyMeasure), W2Pos/1
  DW1/1 -> Cyber/3(DW1)
  M/1 -> Cyber/1(PosW1)
  M1/1 -> Cyber/2(PosW2)
  P1W2/1 -> Cyber/4(P1W2)
  Cyber/2(W2) -> Physical/2(InW2)
  Cyber/1(W1) -> Physical/1(InW1)
  O1/1 -> Cyber/5(OW1)
  O2/1 -> Cyber/6(OW2)
  Physical/1(W1) -> S1/1(PhyMeasure), W1Pos/1
  S1/1(SensorOut) -> M/1

== system c00001M_harness/M172 ==
  DW1 : Inport  OutMin=0  OutMax=4  OutDataTypeStr=int8
  P1W2 : Inport  Port=2  OutMin=0  OutMax=4  OutDataTypeStr=int8
  O1 : Inport  Port=3  OutDataTypeStr=boolean
  O2 : Inport  Port=4  OutDataTypeStr=boolean
  Cyber : Subsystem
  M : Memory
  M1 : Memory
  Physical : Subsystem
  S1 : Subsystem
  S2 : Subsystem
  W1Pos : Outport
  W2Pos : Outport  Port=2
  wires:
  S2/1(SensorOut) -> M1/1
  Physical/2(W2) -> S2/1(PhyMeasure), W2Pos/1
  DW1/1 -> Cyber/3(DW1)
  M/1 -> Cyber/1(PosW1)
  M1/1 -> Cyber/2(PosW2)
  P1W2/1 -> Cyber/4(P1W2)
  Cyber/2(W2) -> Physical/2(InW2)
  Cyber/1(W1) -> Physical/1(InW1)
  O1/1 -> Cyber/5(OW1)
  O2/1 -> Cyber/6(OW2)
  Physical/1(W1) -> S1/1(PhyMeasure), W1Pos/1
  S1/1(SensorOut) -> M/1

== system c00001M_harness/CPSUT/Cyber ==
  note: D = Driver (W1)
      | P1 = Passenger 1 (W2)
      | P2 = Passenger 2 (W3)
      | P3 = Passenger 3 (W4)
      | O = Obstacle
      | C = Control
      | Pri = Prioritizer
      | LD = LockDriver
      | PosW = PositionWindow
      | WL = WindowLogic
      | OW = ObstacleWindow
      | CWXC = ControlWindowXCentralized
      | S = Sensor
      | L = Lock
      | WPos = WindowPosition
      | M = Memory
      | InW = InputWindow
      | WIn = WindowInput
  note: 1: SUBE
      | 0: PARADO
      | -1 BAJA
  note: USERS
      | ---------------------------------
      | 0: None
      | 1: Ventana Arriba
      | 2: Ventana hasta arriba
      | 3: Ventana abajo
      | 4: Ventana hasta abajo
  note: Sensors
  note: Users
  note: Sensors
  note: Users
  note: Sensors
  note: Users
  note: Users
  note: Inputs for window 4
  note: Inputs for window 3
  note: Inputs for Window 2
  note: Inputs For Window1
  note: Sensors
  PosW1 : Inport
  PosW2 : Inport  Port=2
  DW1 : Inport  Port=3
  P1W2 : Inport  Port=4
  OW1 : Inport  Port=5
  OW2 : Inport  Port=6
  WL : Subsystem
  WL1 : Subsystem
  W1 : Outport
  W2 : Outport  Port=2
  wires:
  PosW1/1 -> WL/1(WPos)
  OW1/1 -> WL/3(OW)
  WL/1(WindowLogicOutput) -> W1/1
  PosW2/1 -> WL1/1(WPos)
  OW2/1 -> WL1/3(OW)
  WL1/1(WindowLogicOutput) -> W2/1
  DW1/1 -> WL/2(User)
  P1W2/1 -> WL1/2(User)

== system c00001M_harness/CPSUT/Physical ==
  InW1 : Inport
  InW2 : Inport  Port=2
  W : Subsystem
  W5 : Subsystem
  W1 : Outport
  W2 : Outport  Port=2
  wires:
  InW1/1 -> W/1(WIn)
  InW2/1 -> W5/1(WIn)
  W/1(WPos) -> W1/1
  W5/1(WPos) -> W2/1

== system c00001M_harness/CPSUT/S1 ==
  PhyMeasure : Inport
  SensorOut : Outport
  wires:
  PhyMeasure/1 -> SensorOut/1

== system c00001M_harness/CPSUT/S2 ==
  PhyMeasure : Inport
  SensorOut : Outport
  wires:
  PhyMeasure/1 -> SensorOut/1

== system c00001M_harness/M001/Cyber ==
  note: D = Driver (W1)
      | P1 = Passenger 1 (W2)
      | P2 = Passenger 2 (W3)
      | P3 = Passenger 3 (W4)
      | O = Obstacle
      | C = Control
      | Pri = Prioritizer
      | LD = LockDriver
      | PosW = PositionWindow
      | WL = WindowLogic
      | OW = ObstacleWindow
      | CWXC = ControlWindowXCentralized
      | S = Sensor
      | L = Lock
      | WPos = WindowPosition
      | M = Memory
      | InW = InputWindow
      | WIn = WindowInput
  note: 1: SUBE
      | 0: PARADO
      | -1 BAJA
  note: USERS
      | ---------------------------------
      | 0: None
      | 1: Ventana Arriba
      | 2: Ventana hasta arriba
      | 3: Ventana abajo
      | 4: Ventana hasta abajo
  note: Sensors
  note: Users
  note: Sensors
  note: Users
  note: Sensors
  note: Users
  note: Users
  note: Inputs for window 4
  note: Inputs for window 3
  note: Inputs for Window 2
  note: Inputs For Window1
  note: Sensors
  PosW1 : Inport
  PosW2 : Inport  Port=2
  DW1 : Inport  Port=3
  P1W2 : Inport  Port=4
  OW1 : Inport  Port=5
  OW2 : Inport  Port=6
  WL : Subsystem
  WL1 : Subsystem
  W1 : Outport
  W2 : Outport  Port=2
  wires:
  PosW1/1 -> WL/1(WPos)
  OW1/1 -> WL/3(OW)
  WL/1(WindowLogicOutput) -> W1/1
  PosW2/1 -> WL1/1(WPos)
  OW2/1 -> WL1/3(OW)
  WL1/1(WindowLogicOutput) -> W2/1
  DW1/1 -> WL/2(User)
  P1W2/1 -> WL1/2(User)

== system c00001M_harness/M001/Physical ==
  InW1 : Inport
  InW2 : Inport  Port=2
  W : Subsystem
  W5 : Subsystem
  W1 : Outport
  W2 : Outport  Port=2
  wires:
  InW1/1 -> W/1(WIn)
  InW2/1 -> W5/1(WIn)
  W/1(WPos) -> W1/1
  W5/1(WPos) -> W2/1

== system c00001M_harness/M001/S1 ==
  PhyMeasure : Inport
  SensorOut : Outport
  wires:
  PhyMeasure/1 -> SensorOut/1

== system c00001M_harness/M001/S2 ==
  PhyMeasure : Inport
  SensorOut : Outport
  wires:
  PhyMeasure/1 -> SensorOut/1

== system c00001M_harness/M002/Cyber ==
  note: Sensors
  note: Inputs For Window1
  note: Inputs for Window 2
  note: Inputs for window 3
  note: Inputs for window 4
  note: Users
  note: Users
  note: Sensors
  note: Users
  note: Sensors
  note: Users
  note: Sensors
  note: USERS
      | ---------------------------------
      | 0: None
      | 1: Ventana Arriba
      | 2: Ventana hasta arriba
      | 3: Ventana abajo
      | 4: Ventana hasta abajo
  note: 1: SUBE
      | 0: PARADO
      | -1 BAJA
  note: D = Driver (W1)
      | P1 = Passenger 1 (W2)
      | P2 = Passenger 2 (W3)
      | P3 = Passenger 3 (W4)
      | O = Obstacle
      | C = Control
      | Pri = Prioritizer
      | LD = LockDriver
      | PosW = PositionWindow
      | WL = WindowLogic
      | OW = ObstacleWindow
      | CWXC = ControlWindowXCentralized
      | S = Sensor
      | L = Lock
      | WPos = WindowPosition
      | M = Memory
      | InW = InputWindow
      | WIn = WindowInput
  PosW1 : Inport
  PosW2 : Inport  Port=2
  DW1 : Inport  Port=3
  P1W2 : Inport  Port=4
  OW1 : Inport  Port=5
  OW2 : Inport  Port=6
  WL : Subsystem
  WL1 : Subsystem
  W1 : Outport
  W2 : Outport  Port=2
  wires:
  WL1/1(WindowLogicOutput) -> W2/1
  OW2/1 -> WL1/3(OW)
  PosW2/1 -> WL1/1(WPos)
  WL/1(WindowLogicOutput) -> W1/1
  OW1/1 -> WL/3(OW)
  PosW1/1 -> WL/1(WPos)
  DW1/1 -> WL/2(User)
  P1W2/1 -> WL1/2(User)

== system c00001M_harness/M002/Physical ==
  InW1 : Inport
  InW2 : Inport  Port=2
  W : Subsystem
  W5 : Subsystem
  W1 : Outport
  W2 : Outport  Port=2
  wires:
  W5/1(WPos) -> W2/1
  W/1(WPos) -> W1/1
  InW2/1 -> W5/1(WIn)
  InW1/1 -> W/1(WIn)

== system c00001M_harness/M002/S1 ==
  PhyMeasure : Inport
  SensorOut : Outport
  wires:
  PhyMeasure/1 -> SensorOut/1

== system c00001M_harness/M002/S2 ==
  PhyMeasure : Inport
  SensorOut : Outport
  wires:
  PhyMeasure/1 -> SensorOut/1

== system c00001M_harness/M003/Cyber ==
  note: Sensors
  note: Inputs For Window1
  note: Inputs for Window 2
  note: Inputs for window 3
  note: Inputs for window 4
  note: Users
  note: Users
  note: Sensors
  note: Users
  note: Sensors
  note: Users
  note: Sensors
  note: USERS
      | ---------------------------------
      | 0: None
      | 1: Ventana Arriba
      | 2: Ventana hasta arriba
      | 3: Ventana abajo
      | 4: Ventana hasta abajo
  note: 1: SUBE
      | 0: PARADO
      | -1 BAJA
  note: D = Driver (W1)
      | P1 = Passenger 1 (W2)
      | P2 = Passenger 2 (W3)
      | P3 = Passenger 3 (W4)
      | O = Obstacle
      | C = Control
      | Pri = Prioritizer
      | LD = LockDriver
      | PosW = PositionWindow
      | WL = WindowLogic
      | OW = ObstacleWindow
      | CWXC = ControlWindowXCentralized
      | S = Sensor
      | L = Lock
      | WPos = WindowPosition
      | M = Memory
      | InW = InputWindow
      | WIn = WindowInput
  PosW1 : Inport
  PosW2 : Inport  Port=2
  DW1 : Inport  Port=3
  P1W2 : Inport  Port=4
  OW1 : Inport  Port=5
  OW2 : Inport  Port=6
  WL : Subsystem
  WL1 : Subsystem
  W1 : Outport
  W2 : Outport  Port=2
  wires:
  WL1/1(WindowLogicOutput) -> W2/1
  OW2/1 -> WL1/3(OW)
  PosW2/1 -> WL1/1(WPos)
  WL/1(WindowLogicOutput) -> W1/1
  OW1/1 -> WL/3(OW)
  PosW1/1 -> WL/1(WPos)
  DW1/1 -> WL/2(User)
  P1W2/1 -> WL1/2(User)

== system c00001M_harness/M003/Physical ==
  InW1 : Inport
  InW2 : Inport  Port=2
  W : Subsystem
  W5 : Subsystem
  W1 : Outport
  W2 : Outport  Port=2
  wires:
  W5/1(WPos) -> W2/1
  W/1(WPos) -> W1/1
  InW2/1 -> W5/1(WIn)
  InW1/1 -> W/1(WIn)

== system c00001M_harness/M003/S1 ==
  PhyMeasure : Inport
  SensorOut : Outport
  wires:
  PhyMeasure/1 -> SensorOut/1

== system c00001M_harness/M003/S2 ==
  PhyMeasure : Inport
  SensorOut : Outport
  wires:
  PhyMeasure/1 -> SensorOut/1

== system c00001M_harness/M004/Cyber ==
  note: Sensors
  note: Inputs For Window1
  note: Inputs for Window 2
  note: Inputs for window 3
  note: Inputs for window 4
  note: Users
  note: Users
  note: Sensors
  note: Users
  note: Sensors
  note: Users
  note: Sensors
  note: USERS
      | ---------------------------------
      | 0: None
      | 1: Ventana Arriba
      | 2: Ventana hasta arriba
      | 3: Ventana abajo
      | 4: Ventana hasta abajo
  note: 1: SUBE
      | 0: PARADO
      | -1 BAJA
  note: D = Driver (W1)
      | P1 = Passenger 1 (W2)
      | P2 = Passenger 2 (W3)
      | P3 = Passenger 3 (W4)
      | O = Obstacle
      | C = Control
      | Pri = Prioritizer
      | LD = LockDriver
      | PosW = PositionWindow
      | WL = WindowLogic
      | OW = ObstacleWindow
      | CWXC = ControlWindowXCentralized
      | S = Sensor
      | L = Lock
      | WPos = WindowPosition
      | M = Memory
      | InW = InputWindow
      | WIn = WindowInput
  PosW1 : Inport
  PosW2 : Inport  Port=2
  DW1 : Inport  Port=3
  P1W2 : Inport  Port=4
  OW1 : Inport  Port=5
  OW2 : Inport  Port=6
  WL : Subsystem
  WL1 : Subsystem
  W1 : Outport
  W2 : Outport  Port=2
  wires:
  WL1/1(WindowLogicOutput) -> W2/1
  OW2/1 -> WL1/3(OW)
  PosW2/1 -> WL1/1(WPos)
  WL/1(WindowLogicOutput) -> W1/1
  OW1/1 -> WL/3(OW)
  PosW1/1 -> WL/1(WPos)
  DW1/1 -> WL/2(User)
  P1W2/1 -> WL1/2(User)

== system c00001M_harness/M004/Physical ==
  InW1 : Inport
  InW2 : Inport  Port=2
  W : Subsystem
  W5 : Subsystem
  W1 : Outport
  W2 : Outport  Port=2
  wires:
  W5/1(WPos) -> W2/1
  W/1(WPos) -> W1/1
  InW2/1 -> W5/1(WIn)
  InW1/1 -> W/1(WIn)

== system c00001M_harness/M004/S1 ==
  PhyMeasure : Inport
  SensorOut : Outport
  wires:
  PhyMeasure/1 -> SensorOut/1

== system c00001M_harness/M004/S2 ==
  PhyMeasure : Inport
  SensorOut : Outport
  wires:
  PhyMeasure/1 -> SensorOut/1

== system c00001M_harness/M011/Cyber ==
  note: Sensors
  note: Inputs For Window1
  note: Inputs for Window 2
  note: Inputs for window 3
  note: Inputs for window 4
  note: Users
  note: Users
  note: Sensors
  note: Users
  note: Sensors
  note: Users
  note: Sensors
  note: USERS
      | ---------------------------------
      | 0: None
      | 1: Ventana Arriba
      | 2: Ventana hasta arriba
      | 3: Ventana abajo
      | 4: Ventana hasta abajo
  note: 1: SUBE
      | 0: PARADO
      | -1 BAJA
  note: D = Driver (W1)
      | P1 = Passenger 1 (W2)
      | P2 = Passenger 2 (W3)
      | P3 = Passenger 3 (W4)
      | O = Obstacle
      | C = Control
      | Pri = Prioritizer
      | LD = LockDriver
      | PosW = PositionWindow
      | WL = WindowLogic
      | OW = ObstacleWindow
      | CWXC = ControlWindowXCentralized
      | S = Sensor
      | L = Lock
      | WPos = WindowPosition
      | M = Memory
      | InW = InputWindow
      | WIn = WindowInput
  PosW1 : Inport
  PosW2 : Inport  Port=2
  DW1 : Inport  Port=3
  P1W2 : Inport  Port=4
  OW1 : Inport  Port=5
  OW2 : Inport  Port=6
  WL : Subsystem
  WL1 : Subsystem
  W1 : Outport
  W2 : Outport  Port=2
  wires:
  WL1/1(WindowLogicOutput) -> W2/1
  OW2/1 -> WL1/3(OW)
  PosW2/1 -> WL1/1(WPos)
  WL/1(WindowLogicOutput) -> W1/1
  OW1/1 -> WL/3(OW)
  PosW1/1 -> WL/1(WPos)
  DW1/1 -> WL/2(User)
  P1W2/1 -> WL1/2(User)

== system c00001M_harness/M011/Physical ==
  InW1 : Inport
  InW2 : Inport  Port=2
  W : Subsystem
  W5 : Subsystem
  W1 : Outport
  W2 : Outport  Port=2
  wires:
  W5/1(WPos) -> W2/1
  W/1(WPos) -> W1/1
  InW2/1 -> W5/1(WIn)
  InW1/1 -> W/1(WIn)

== system c00001M_harness/M011/S1 ==
  PhyMeasure : Inport
  Add : Sum
  Constant : Constant
  SensorOut : Outport
  wires:
  PhyMeasure/1 -> Add/2
  Add/1 -> SensorOut/1
  Constant/1 -> Add/1

== system c00001M_harness/M011/S2 ==
  PhyMeasure : Inport
  SensorOut : Outport
  wires:
  PhyMeasure/1 -> SensorOut/1

== system c00001M_harness/M012/Cyber ==
  note: Sensors
  note: Inputs For Window1
  note: Inputs for Window 2
  note: Inputs for window 3
  note: Inputs for window 4
  note: Users
  note: Users
  note: Sensors
  note: Users
  note: Sensors
  note: Users
  note: Sensors
  note: USERS
      | ---------------------------------
      | 0: None
      | 1: Ventana Arriba
      | 2: Ventana hasta arriba
      | 3: Ventana abajo
      | 4: Ventana hasta abajo
  note: 1: SUBE
      | 0: PARADO
      | -1 BAJA
  note: D = Driver (W1)
      | P1 = Passenger 1 (W2)
      | P2 = Passenger 2 (W3)
      | P3 = Passenger 3 (W4)
      | O = Obstacle
      | C = Control
      | Pri = Prioritizer
      | LD = LockDriver
      | PosW = PositionWindow
      | WL = WindowLogic
      | OW = ObstacleWindow
      | CWXC = ControlWindowXCentralized
      | S = Sensor
      | L = Lock
      | WPos = WindowPosition
      | M = Memory
      | InW = InputWindow
      | WIn = WindowInput
  PosW1 : Inport
  PosW2 : Inport  Port=2
  DW1 : Inport  Port=3
  P1W2 : Inport  Port=4
  OW1 : Inport  Port=5
  OW2 : Inport  Port=6
  WL : Subsystem
  WL1 : Subsystem
  W1 : Outport
  W2 : Outport  Port=2
  wires:
  WL1/1(WindowLogicOutput) -> W2/1
  OW2/1 -> WL1/3(OW)
  PosW2/1 -> WL1/1(WPos)
  WL/1(WindowLogicOutput) -> W1/1
  OW1/1 -> WL/3(OW)
  PosW1/1 -> WL/1(WPos)
  DW1/1 -> WL/2(User)
  P1W2/1 -> WL1/2(User)

== system c00001M_harness/M012/Physical ==
  InW1 : Inport
  InW2 : Inport  Port=2
  W : Subsystem
  W5 : Subsystem
  W1 : Outport
  W2 : Outport  Port=2
  wires:
  W5/1(WPos) -> W2/1
  W/1(WPos) -> W1/1
  InW2/1 -> W5/1(WIn)
  InW1/1 -> W/1(WIn)

== system c00001M_harness/M012/S1 ==
  PhyMeasure : Inport
  SensorOut : Outport
  wires:
  PhyMeasure/1 -> SensorOut/1

== system c00001M_harness/M012/S2 ==
  PhyMeasure : Inport
  Add : Sum
  Constant : Constant
  SensorOut : Outport
  wires:
  PhyMeasure/1 -> Add/2
  Constant/1 -> Add/1
  Add/1 -> SensorOut/1

== system c00001M_harness/M015/Cyber ==
  note: Sensors
  note: Inputs For Window1
  note: Inputs for Window 2
  note: Inputs for window 3
  note: Inputs for window 4
  note: Users
  note: Users
  note: Sensors
  note: Users
  note: Sensors
  note: Users
  note: Sensors
  note: USERS
      | ---------------------------------
      | 0: None
      | 1: Ventana Arriba
      | 2: Ventana hasta arriba
      | 3: Ventana abajo
      | 4: Ventana hasta abajo
  note: 1: SUBE
      | 0: PARADO
      | -1 BAJA
  note: D = Driver (W1)
      | P1 = Passenger 1 (W2)
      | P2 = Passenger 2 (W3)
      | P3 = Passenger 3 (W4)
      | O = Obstacle
      | C = Control
      | Pri = Prioritizer
      | LD = LockDriver
      | PosW = PositionWindow
      | WL = WindowLogic
      | OW = ObstacleWindow
      | CWXC = ControlWindowXCentralized
      | S = Sensor
      | L = Lock
      | WPos = WindowPosition
      | M = Memory
      | InW = InputWindow
      | WIn = WindowInput
  PosW1 : Inport
  PosW2 : Inport  Port=2
  DW1 : Inport  Port=3
  P1W2 : Inport  Port=4
  OW1 : Inport  Port=5
  OW2 : Inport  Port=6
  WL : Subsystem
  WL1 : Subsystem
  W1 : Outport
  W2 : Outport  Port=2
  wires:
  WL1/1(WindowLogicOutput) -> W2/1
  OW2/1 -> WL1/3(OW)
  PosW2/1 -> WL1/1(WPos)
  WL/1(WindowLogicOutput) -> W1/1
  OW1/1 -> WL/3(OW)
  PosW1/1 -> WL/1(WPos)
  DW1/1 -> WL/2(User)
  P1W2/1 -> WL1/2(User)

== system c00001M_harness/M015/Physical ==
  InW1 : Inport
  InW2 : Inport  Port=2
  W : Subsystem
  W5 : Subsystem
  W1 : Outport
  W2 : Outport  Port=2
  wires:
  W5/1(WPos) -> W2/1
  W/1(WPos) -> W1/1
  InW2/1 -> W5/1(WIn)
  InW1/1 -> W/1(WIn)

== system c00001M_harness/M015/S1 ==
  PhyMeasure : Inport
  SensorOut : Outport
  wires:
  PhyMeasure/1 -> SensorOut/1

== system c00001M_harness/M015/S2 ==
  PhyMeasure : Inport
  SensorOut : Outport
  wires:
  PhyMeasure/1 -> SensorOut/1

== system c00001M_harness/M016/Cyber ==
  note: Sensors
  note: Inputs For Window1
  note: Inputs for Window 2
  note: Inputs for window 3
  note: Inputs for window 4
  note: Users
  note: Users
  note: Sensors
  note: Users
  note: Sensors
  note: Users
  note: Sensors
  note: USERS
      | ---------------------------------
      | 0: None
      | 1: Ventana Arriba
      | 2: Ventana hasta arriba
      | 3: Ventana abajo
      | 4: Ventana hasta abajo
  note: 1: SUBE
      | 0: PARADO
      | -1 BAJA
  note: D = Driver (W1)
      | P1 = Passenger 1 (W2)
      | P2 = Passenger 2 (W3)
      | P3 = Passenger 3 (W4)
      | O = Obstacle
      | C = Control
      | Pri = Prioritizer
      | LD = LockDriver
      | PosW = PositionWindow
      | WL = WindowLogic
      | OW = ObstacleWindow
      | CWXC = ControlWindowXCentralized
      | S = Sensor
      | L = Lock
      | WPos = WindowPosition
      | M = Memory
      | InW = InputWindow
      | WIn = WindowInput
  PosW1 : Inport
  PosW2 : Inport  Port=2
  DW1 : Inport  Port=3
  P1W2 : Inport  Port=4
  OW1 : Inport  Port=5
  OW2 : Inport  Port=6
  WL : Subsystem
  WL1 : Subsystem
  W1 : Outport
  W2 : Outport  Port=2
  wires:
  WL1/1(WindowLogicOutput) -> W2/1
  OW2/1 -> WL1/3(OW)
  PosW2/1 -> WL1/1(WPos)
  WL/1(WindowLogicOutput) -> W1/1
  OW1/1 -> WL/3(OW)
  PosW1/1 -> WL/1(WPos)
  DW1/1 -> WL/2(User)
  P1W2/1 -> WL1/2(User)

== system c00001M_harness/M016/Physical ==
  InW1 : Inport
  InW2 : Inport  Port=2
  W : Subsystem
  W5 : Subsystem
  W1 : Outport
  W2 : Outport  Port=2
  wires:
  W5/1(WPos) -> W2/1
  W/1(WPos) -> W1/1
  InW2/1 -> W5/1(WIn)
  InW1/1 -> W/1(WIn)

== system c00001M_harness/M016/S1 ==
  PhyMeasure : Inport
  SensorOut : Outport
  wires:
  PhyMeasure/1 -> SensorOut/1

== system c00001M_harness/M016/S2 ==
  PhyMeasure : Inport
  SensorOut : Outport
  wires:
  PhyMeasure/1 -> SensorOut/1
